simulink model "pid_exercise"  (R2018a)
settings: Solver=VariableStepAuto  StartTime=0.0  StopTime=20.0  RelTol=1e-3
values from neighbouring files (symbols this model uses):
  cc = 0.1    [param1.m]    (also in param2.m)
  Kp = 735    [notebook.m]    (also in param1.m = 5; param2.m = 10)
  m = 1.0    (= 1)    [param1.m]    (also in param2.m)
  T = 0.01    [param1.m]    (also in param2.m)
  tau = 1.0e-3    (= 0.001)    [param1.m]    (also in param2.m)
  tau_d = 4.5    [param1.m]    (also in param2.m = 0.1)
  tau_i = 20    [param1.m]    (also in param2.m)
settings Model: Creator=mamoru  LastModifiedBy=mamoru

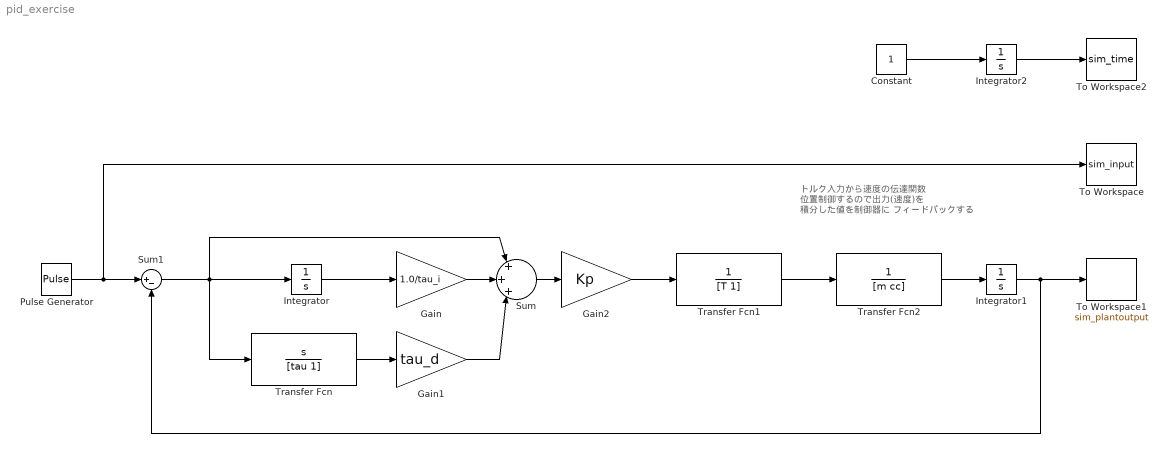
== system pid_exercise ==
  note: トルク入力から速度の伝達関数
      | 位置制御するので出力(速度)を
      | 積分した値を制御器に
      | フィードバックする
  Constant : Constant
  Gain : Gain  Gain=1.0/tau_i
  Gain1 : Gain  Gain=tau_d
  Gain2 : Gain  Gain=Kp
  Integrator : Integrator
  Integrator1 : Integrator
  Integrator2 : Integrator
  Pulse Generator : DiscretePulseGenerator  PulseType=Time based  Period=10  PulseWidth=50
  Sum : Sum  Inputs=|+|+|+|
  Sum1 : Sum  Inputs=|+-
  To Workspace : ToWorkspace  VariableName=sim_input  SampleTime=-1
      settings: Save2DSignal=2-D array (concatenate along first dimension)
  To Workspace1 : ToWorkspace  VariableName=sim_plantoutput  SampleTime=-1
      settings: Save2DSignal=2-D array (concatenate along first dimension)
  To Workspace2 : ToWorkspace  VariableName=sim_time  SampleTime=-1
      settings: Save2DSignal=2-D array (concatenate along first dimension)
  Transfer Fcn : TransferFcn  Numerator=[1 0]  Denominator=[tau 1]
  Transfer Fcn1 : TransferFcn  Denominator=[T 1]
  Transfer Fcn2 : TransferFcn  Denominator=[m cc]
  wires:
  Integrator/1 -> Gain/1
  Transfer Fcn/1 -> Gain1/1
  Sum/1 -> Gain2/1
  Gain/1 -> Sum/2
  Pulse Generator/1 -> To Workspace/1, Sum1/1
  Sum1/1 -> Sum/1, Transfer Fcn/1, Integrator/1
  Gain1/1 -> Sum/3
  Gain2/1 -> Transfer Fcn1/1
  Transfer Fcn1/1 -> Transfer Fcn2/1
  Integrator1/1 -> To Workspace1/1, Sum1/2
  Transfer Fcn2/1 -> Integrator1/1
  Integrator2/1 -> To Workspace2/1
  Constant/1 -> Integrator2/1
